simulink model "Simulation_3D_LQR"  (R2016b)
settings: Solver=FixedStepAuto  StartTime=0.0  StopTime=30  FixedStep=0.001  RelTol=1e-3
undefined symbols (not defined in the file or in its folder): A, B, F_final, x_0
libraries: simulink x1
settings Model: Creator=ich  LastModifiedBy=michael

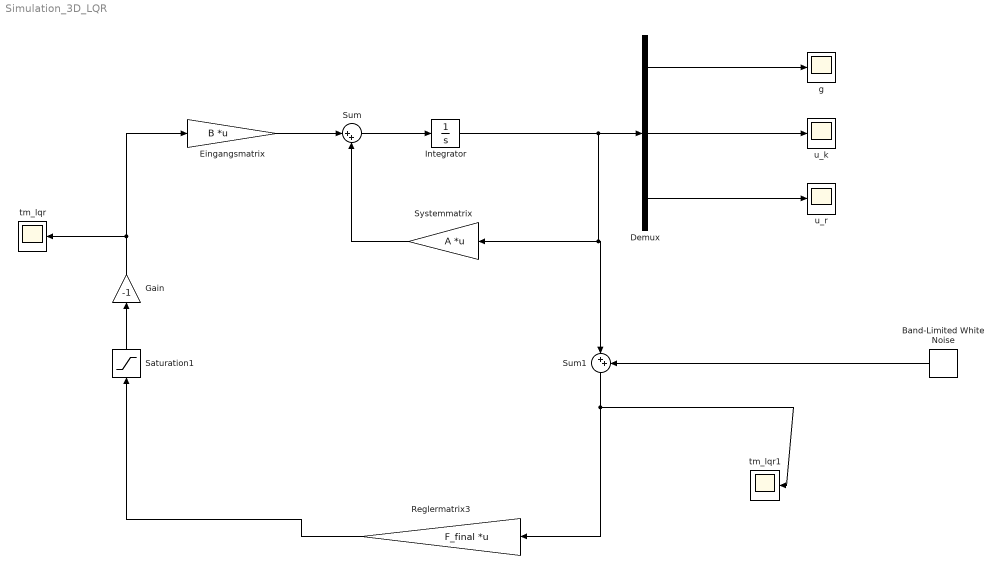
== system Simulation_3D_LQR ==
  Band-Limited White Noise : simulink/Sources/Band-Limited White Noise  Cov=[0.000250;0.000250;0.000250; zeros(6,1)]  Ts=0.001  seed=[23341]
  Demux : Demux  Outputs=3
  Eingangsmatrix : Gain  Gain=B  Multiplication=Matrix(K*u) (u vector)
  Gain : Gain  Gain=-1
  Integrator : Integrator  InitialCondition=x_0
  Reglermatrix3 : Gain  Gain=F_final  Multiplication=Matrix(K*u) (u vector)
  Saturation1 : Saturate  UpperLimit=0.11  LowerLimit=-0.11
  Sum : Sum  Inputs=|++  OutDataTypeStr=double
  Sum1 : Sum  Inputs=|++
  Systemmatrix : Gain  Gain=A  Multiplication=Matrix(K*u) (u vector)
  g : Scope
  tm_lqr : Scope
  tm_lqr1 : Scope
  u_k : Scope
  u_r : Scope
  wires:
  Eingangsmatrix/1 -> Sum/1
  Systemmatrix/1 -> Sum/2
  Gain/1 -> Eingangsmatrix/1, tm_lqr/1
  Sum/1 -> Integrator/1
  Demux/1 -> g/1
  Demux/3 -> u_r/1
  Demux/2 -> u_k/1
  Integrator/1 -> Sum1/1, Systemmatrix/1, Demux/1
  Reglermatrix3/1 -> Saturation1/1
  Saturation1/1 -> Gain/1
  Sum1/1 -> tm_lqr1/1, Reglermatrix3/1
  Band-Limited White Noise/1 -> Sum1/2
